simulink model "task_3_x"  (R2021b)
settings: Solver=FixedStepAuto  StartTime=0.0  StopTime=2  FixedStep=0.00005  RelTol=1e-3
settings Model: Creator=den  LastModifiedBy=den

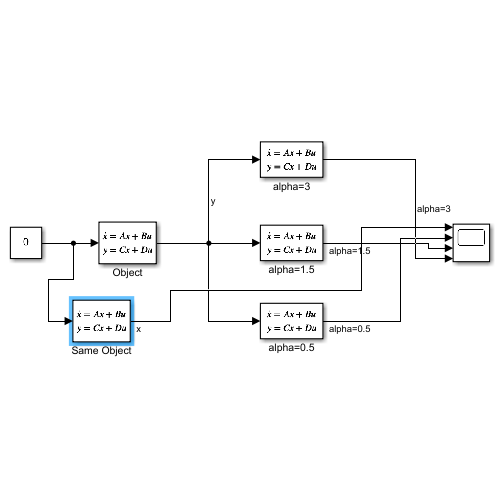
[thumbnail: Simulink's stored preview of the top-level diagram]
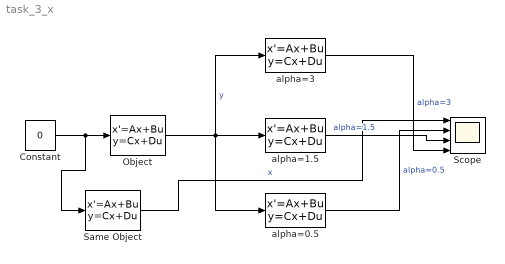
== system task_3_x ==
  Constant : Constant  Value=0
  Object : StateSpace  A=[0 5 0 0; -5 0 0 0; 0 0 0 1; 0 0 -1 0]  B=[0; 0; 0; 0]  C=[0 9 1 0]  D=0  InitialCondition=[-3; 17; 2; -8]
  Same Object : StateSpace  A=[0 5 0 0; -5 0 0 0; 0 0 0 1; 0 0 -1 0]  B=[0; 0; 0; 0]  C=[1 0 0 0; 0 1 0 0; 0 0 1 0; 0 0 0 1]  D=[0;0;0;0]  InitialCondition=[-3; 17; 2; -8]
  Scope : Scope  NumInputPorts=4
  alpha=0.5 : StateSpace  A="[    0   20.9943    1.7771         0;   -5.0000    0.0606    0.0067         0;   0  -52.5686   -5.8410    1.0000;     0  -22.1377   -3.4597         0]"  B=|  C=[1 0 0 0; 0 1 0 0; 0 0 1 0; 0 0 0 1]  D=[0;0;0;0]  InitialCondition=[5; 1; -9; 11]
      | [
      |    -1.7771
      |  ;  -0.0067
      |    ; 5.8410
      |   ;  2.4597]
  alpha=1.5 : StateSpace  A=|  B=|  C=[1 0 0 0; 0 1 0 0; 0 0 1 0; 0 0 0 1]  D=[0;0;0;0]  InitialCondition=[5; 1; -9; 11]
      A=|
      | [0   47.5325    4.7258         0; -5.0000   23.4331    2.6037         0;  0 -363.0978  -40.3442    1.0000; 0 -409.3974  -46.4886         0
      | ]
      B=|
      | [   -4.7258
      |  ;  -2.6037
      |  ;  40.3442
      |    ;45.4886]
  alpha=3 : StateSpace  A="1.0e+03*[0    0.0501    0.0050         0; -0.0050    0.0892    0.0099         0; 0   -1.0418   -0.1158    0.0010;0   -2.0312   -0.2267         0]"  B=|  C=[1 0 0 0; 0 1 0 0; 0 0 1 0; 0 0 0 1]  D=[0;0;0;0]  InitialCondition=[5; 1; -9; 11]
      | [   -5.0057;
      |    -9.9057
      | ;  115.7500;
      |   225.6841]
  wires:
  Object/1 -> alpha=0.5/1, alpha=1.5/1, alpha=3/1  "y"
  alpha=3/1 -> Scope/4  "alpha=3"
  Constant/1 -> Same Object/1, Object/1
  alpha=1.5/1 -> Scope/3  "alpha=1.5"
  alpha=0.5/1 -> Scope/2  "alpha=0.5"
  Same Object/1 -> Scope/1  "x"
